simulink subsystem "Write_ULOG_Data"  (R2025a)
settings: Solver=VariableStepAuto  StartTime=0.0  StopTime=10.0  RelTol=1e-3
libraries: px4Utilslib x2
settings Model: Creator=gurt1  LastModifiedBy=gurt1
settings RTWCC: GPUComputeCapability=3.5

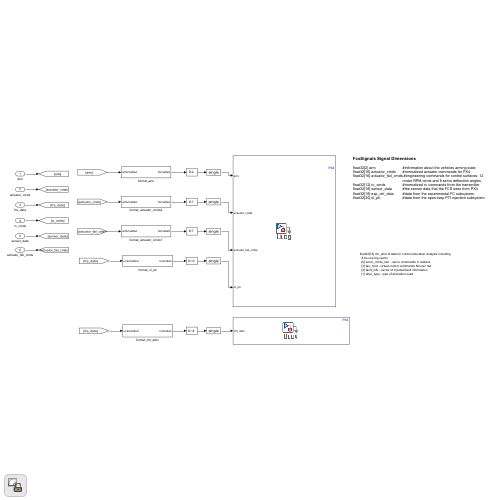
[thumbnail: Simulink's stored preview of the top-level diagram]
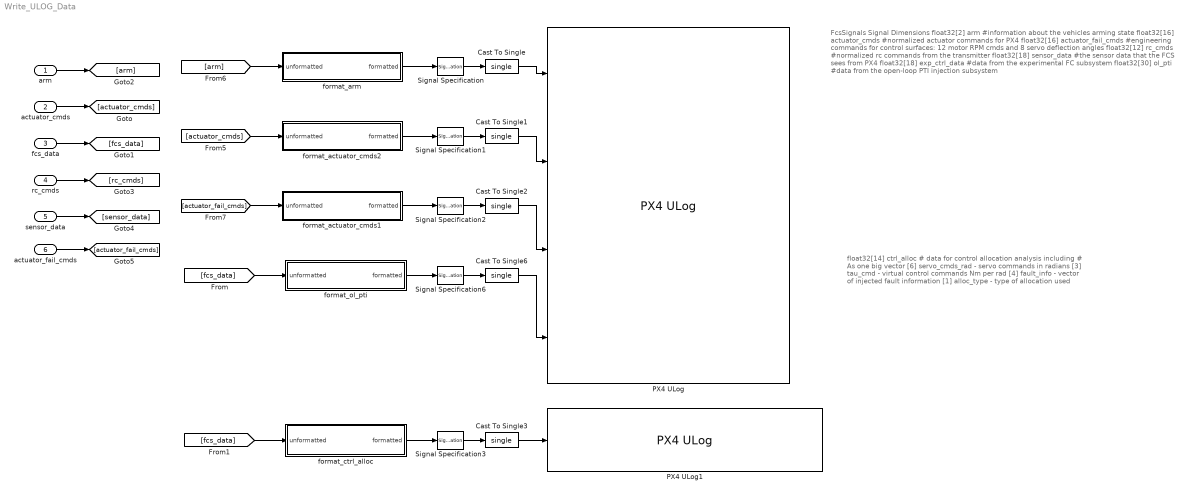
== system Write_ULOG_Data ==
  note: float32[14] ctrl_alloc # data for control allocation analysis including
      |   # As one big vector
      |   [6] servo_cmds_rad  - servo commands in radians
      |   [3] tau_cmd - virtual control commands Nm per rad
      |   [4] fault_info - vector of injected fault information
      |   [1] alloc_type - type of allocation used
  note: FcsSignals Signal Dimensions
      |
      | float32[2] arm #information about the vehicles arming state
      | float32[16] actuator_cmds #normalized actuator commands for PX4
      | float32[16] actuator_fail_cmds #engineering commands for control surfaces: 12 motor RPM cmds and 8 servo deflection angles
      | float32[12] rc_cmds #normalized rc commands from the transmitter
      | float32[18] sensor_data #the sensor data that the FCS sees from PX4
      | float32[18] exp_ctrl_data #data from the experimental FC subsystem
      | float32[30] ol_pti #data from the open-loop PTI injection subsystem
  arm : Inport
  actuator_cmds : Inport  Port=2
  fcs_data : Inport  Port=3
  rc_cmds : Inport  Port=4
  sensor_data : Inport  Port=5
  actuator_fail_cmds : Inport  Port=6
  Cast To Single{,1..3,6} (5 alike) : DataTypeConversion  OutDataTypeStr=single  SaturateOnIntegerOverflow=off  RndMeth=Floor
  PX4 ULog : px4Utilslib/PX4 ULog  uORBTopic=FcsSignals
  PX4 ULog1 : px4Utilslib/PX4 ULog  uORBTopic=CaSignals
  Signal Specification : SignalSpecification  Dimensions=2
  Signal Specification1 : SignalSpecification  Dimensions=7
  Signal Specification2 : SignalSpecification  Dimensions=7
  Signal Specification3 : SignalSpecification  Dimensions=14
  Signal Specification6 : SignalSpecification  Dimensions=10
  format_actuator_cmds1 : Subsystem
  format_actuator_cmds2 : Subsystem
  format_arm : Subsystem
  format_ctrl_alloc : Subsystem
  format_ol_pti : Subsystem
  wires:
  actuator_cmds/1 -> [actuator_cmds]
  arm/1 -> [arm]
  fcs_data/1 -> [fcs_data]
  sensor_data/1 -> [sensor_data]
  rc_cmds/1 -> [rc_cmds]
  [fcs_data] -> format_ol_pti/1(unformatted)
  [actuator_fail_cmds] -> format_actuator_cmds1/1(unformatted)
  format_actuator_cmds2/1(formatted) -> Signal Specification1/1
  format_arm/1(formatted) -> Signal Specification/1
  [actuator_cmds] -> format_actuator_cmds2/1(unformatted)
  [arm] -> format_arm/1(unformatted)
  format_ol_pti/1(formatted) -> Signal Specification6/1
  Signal Specification/1 -> Cast To Single/1
  Signal Specification1/1 -> Cast To Single1/1
  Signal Specification2/1 -> Cast To Single2/1
  Signal Specification6/1 -> Cast To Single6/1
  actuator_fail_cmds/1 -> [actuator_fail_cmds]
  format_actuator_cmds1/1(formatted) -> Signal Specification2/1
  Cast To Single6/1 -> PX4 ULog/4
  Cast To Single/1 -> PX4 ULog/1
  Cast To Single1/1 -> PX4 ULog/2
  Cast To Single2/1 -> PX4 ULog/3
  Cast To Single3/1 -> PX4 ULog1/1
  [fcs_data] -> format_ctrl_alloc/1(unformatted)
  format_ctrl_alloc/1(formatted) -> Signal Specification3/1
  Signal Specification3/1 -> Cast To Single3/1

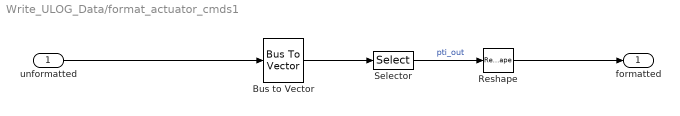
== system Write_ULOG_Data/format_actuator_cmds1 ==
  unformatted : Inport
  Bus to Vector : BusToVector
  Reshape : Reshape
  Selector : Selector  InputPortWidth=16  IndexOptions=Index vector (dialog)  Indices=[1,9:14]  OutputSizes=1
  formatted : Outport
  wires:
  Selector/1 -> Reshape/1  "pti_out"
  unformatted/1 -> Bus to Vector/1
  Reshape/1 -> formatted/1
  Bus to Vector/1 -> Selector/1

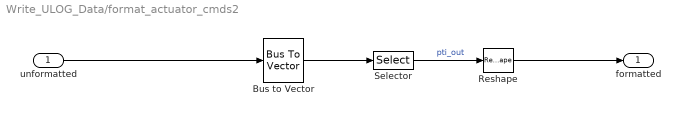
== system Write_ULOG_Data/format_actuator_cmds2 ==
  unformatted : Inport
  Bus to Vector : BusToVector
  Reshape : Reshape
  Selector : Selector  InputPortWidth=16  IndexOptions=Index vector (dialog)  Indices=[1,9:14]  OutputSizes=1
  formatted : Outport
  wires:
  Bus to Vector/1 -> Selector/1
  Reshape/1 -> formatted/1
  unformatted/1 -> Bus to Vector/1
  Selector/1 -> Reshape/1  "pti_out"

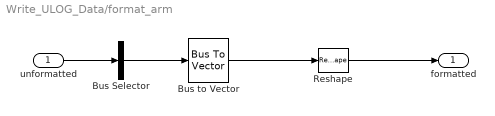
== system Write_ULOG_Data/format_arm ==
  unformatted : Inport
  Bus Selector : BusSelector  OutputSignals=arm,dt_arm  OutputAsBus=on
  Bus to Vector : BusToVector
  Reshape : Reshape
  formatted : Outport
  wires:
  Bus to Vector/1 -> Reshape/1
  unformatted/1 -> Bus Selector/1
  Reshape/1 -> formatted/1
  Bus Selector/1 -> Bus to Vector/1

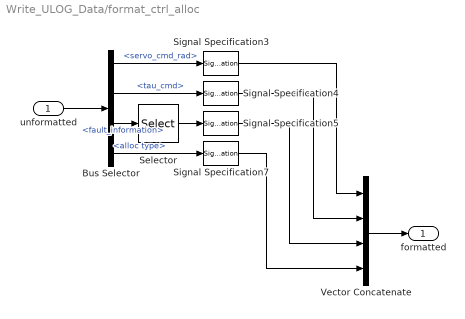
== system Write_ULOG_Data/format_ctrl_alloc ==
  unformatted : Inport
  Bus Selector : BusSelector  OutputSignals=main_CA.servo_cmd_rad,main_CA.tau_cmd,main_CA.fault_information,main_CA.alloc type
  Selector : Selector  InputPortWidth=16  IndexOptions=Index vector (dialog)  Indices=[1:4]  OutputSizes=1
  Signal Specification3 : SignalSpecification  Dimensions=6
  Signal Specification4 : SignalSpecification  Dimensions=3
  Signal Specification5 : SignalSpecification  Dimensions=4
  Signal Specification7 : SignalSpecification  Dimensions=1
  Vector Concatenate : Concatenate  NumInputs=4
  formatted : Outport
  wires:
  Signal Specification7/1 -> Vector Concatenate/4
  Selector/1 -> Signal Specification5/1
  Vector Concatenate/1 -> formatted/1
  Signal Specification4/1 -> Vector Concatenate/2
  Bus Selector/1 -> Signal Specification3/1  "<servo_cmd_rad>"
  Signal Specification3/1 -> Vector Concatenate/1
  Signal Specification5/1 -> Vector Concatenate/3
  Bus Selector/3 -> Selector/1  "<fault_information>"
  Bus Selector/4 -> Signal Specification7/1  "<alloc type>"
  unformatted/1 -> Bus Selector/1
  Bus Selector/2 -> Signal Specification4/1  "<tau_cmd>"

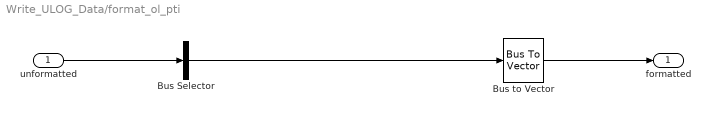
== system Write_ULOG_Data/format_ol_pti ==
  unformatted : Inport
  Bus Selector : BusSelector  OutputSignals=OL_PTI.pti_out,OL_PTI.t_gcs,OL_PTI.pti_ms_amp,OL_PTI.pti_ms_t  OutputAsBus=on
  Bus to Vector : BusToVector
  formatted : Outport
  wires:
  unformatted/1 -> Bus Selector/1
  Bus to Vector/1 -> formatted/1
  Bus Selector/1 -> Bus to Vector/1
